simulink library "asbhl20vehicle"  (R2016b)
settings: Solver=ode45  StartTime=0.0  StopTime=10.0  RelTol=1e-3
undefined symbols (not defined in the file): alpha_vec_Cn0, b_ref, beta_vec_Cn0, Clbeta, Clda, Clddf, Cldr, Clp, Clr, Cm0, cm_GE, cm_LG, Cmda, Cmde, Cmdfn, Cmdfp, Cmdr, Cmq, Cn0, Cnda, Cnddf, Cndr, Cnp, Cnr, CX0, cx_GE, cx_LG, CXda, CXddf, CXde, CXdfn, CXdfp, CXdr, CYbeta, CYda, CYddf, CYdr, CZ0, cz_GE, cz_LG, CZda, CZde, CZdfn, CZdfp, CZdr, d_ref, Earth, Euler_0, heading0, LongLat0, mass, Tfg, Tplant, Ts, WGS84, x_cg, x_ref
libraries: aerolibtransform2 x6, aerolibconvert2 x4, aerolibasang x3, aerolibobsolete x3, aerolibutil x3, aerolib6dof2 x1, aerolibadyn x1, asbhl20act x1, discretizing x1
(part 2 of 2)

== system asbhl20vehicle/Vehicle/Aerodynamic/Aerodynamic Coefficients/Actuator Increments/Flap(pos) ==
  Alpha : Inport
  Actuators : Inport  Port=2
  Bus Selector : BusSelector  OutputSignals=Flap(pos)
  Bus Selector1 : BusSelector  OutputSignals=k,f
  Bus Selector3 : BusSelector  OutputSignals=k,f
  Bus Selector5 : BusSelector  OutputSignals=k,f
  Cm : Interpolation_n-D  NumberOfTableDimensions=1  Table=Cmdfp  RemoveProtectionIndex=on  SaturateOnIntegerOverflow=on
      settings: InputPortMap=u0,u1
  Constant1 : Constant  Value=0
  Constant2 : Constant  Value=0
  Constant3 : Constant  Value=0
  Cx : Interpolation_n-D  NumberOfTableDimensions=1  Table=CXdfp  RemoveProtectionIndex=on  SaturateOnIntegerOverflow=on
      settings: InputPortMap=u0,u1
  Cz : Interpolation_n-D  NumberOfTableDimensions=1  Table=CZdfp  RemoveProtectionIndex=on  SaturateOnIntegerOverflow=on
      settings: InputPortMap=u0,u1
  Mux1 : Mux  Inputs=6
  Product : Product  SaturateOnIntegerOverflow=on  InputSameDT=on  OutDataTypeStr=Inherit: Same as first input
  delCoeff : Outport
  wires:
  Product/1 -> delCoeff/1
  Mux1/1 -> Product/1
  Alpha/1 -> Bus Selector5/1, Bus Selector3/1, Bus Selector1/1
  Cx/1 -> Mux1/1
  Cz/1 -> Mux1/3
  Cm/1 -> Mux1/5
  Constant1/1 -> Mux1/2
  Constant2/1 -> Mux1/4
  Constant3/1 -> Mux1/6
  Actuators/1 -> Bus Selector/1
  Bus Selector/1 -> Product/2  "<Flap(pos)>"
  Bus Selector5/1 -> Cm/1  "<k>"
  Bus Selector5/2 -> Cm/2  "<f>"
  Bus Selector3/1 -> Cz/1  "<k>"
  Bus Selector3/2 -> Cz/2  "<f>"
  Bus Selector1/1 -> Cx/1  "<k>"
  Bus Selector1/2 -> Cx/2  "<f>"

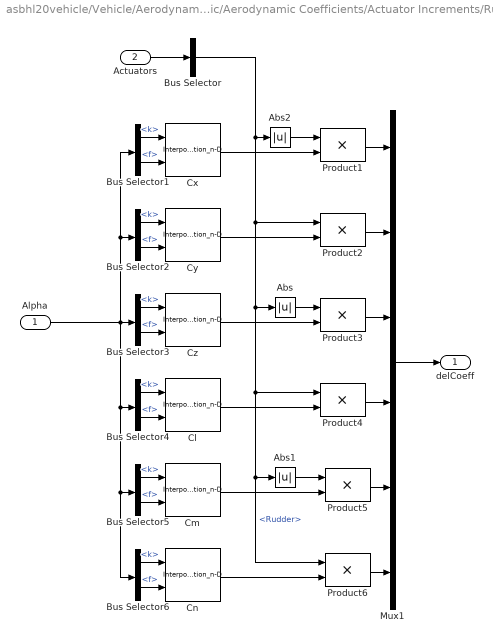
== system asbhl20vehicle/Vehicle/Aerodynamic/Aerodynamic Coefficients/Actuator Increments/Rudder ==
  Alpha : Inport
  Actuators : Inport  Port=2
  Abs : Abs  SaturateOnIntegerOverflow=on
  Abs1 : Abs  SaturateOnIntegerOverflow=on
  Abs2 : Abs  SaturateOnIntegerOverflow=on
  Bus Selector : BusSelector  OutputSignals=Rudder
  Bus Selector{1..6} (6 alike) : BusSelector  OutputSignals=k,f
  Cl : Interpolation_n-D  NumberOfTableDimensions=1  Table=Cldr  RemoveProtectionIndex=on  SaturateOnIntegerOverflow=on
      settings: InputPortMap=u0,u1
  Cm : Interpolation_n-D  NumberOfTableDimensions=1  Table=Cmdr  RemoveProtectionIndex=on  SaturateOnIntegerOverflow=on
      settings: InputPortMap=u0,u1
  Cn : Interpolation_n-D  NumberOfTableDimensions=1  Table=Cndr  RemoveProtectionIndex=on  SaturateOnIntegerOverflow=on
      settings: InputPortMap=u0,u1
  Cx : Interpolation_n-D  NumberOfTableDimensions=1  Table=CXdr  RemoveProtectionIndex=on  SaturateOnIntegerOverflow=on
      settings: InputPortMap=u0,u1
  Cy : Interpolation_n-D  NumberOfTableDimensions=1  Table=CYdr  RemoveProtectionIndex=on  SaturateOnIntegerOverflow=on
      settings: InputPortMap=u0,u1
  Cz : Interpolation_n-D  NumberOfTableDimensions=1  Table=CZdr  RemoveProtectionIndex=on  SaturateOnIntegerOverflow=on
      settings: InputPortMap=u0,u1
  Mux1 : Mux  Inputs=6
  Product{1..6} (6 alike) : Product  SaturateOnIntegerOverflow=on  InputSameDT=on  OutDataTypeStr=Inherit: Same as first input
  delCoeff : Outport
  wires:
  Actuators/1 -> Bus Selector/1
  Mux1/1 -> delCoeff/1
  Product1/1 -> Mux1/1
  Cx/1 -> Product1/2
  Product2/1 -> Mux1/2
  Cy/1 -> Product2/2
  Product3/1 -> Mux1/3
  Cz/1 -> Product3/2
  Cl/1 -> Product4/2
  Product4/1 -> Mux1/4
  Cm/1 -> Product5/2
  Product5/1 -> Mux1/5
  Cn/1 -> Product6/2
  Product6/1 -> Mux1/6
  Bus Selector/1 -> Abs2/1, Product2/1, Abs/1, Product4/1, Abs1/1, Product6/1  "<Rudder>"
  Abs/1 -> Product3/1
  Abs1/1 -> Product5/1
  Abs2/1 -> Product1/1
  Alpha/1 -> Bus Selector3/1, Bus Selector4/1, Bus Selector6/1, Bus Selector5/1, Bus Selector2/1, Bus Selector1/1
  Bus Selector1/1 -> Cx/1  "<k>"
  Bus Selector1/2 -> Cx/2  "<f>"
  Bus Selector2/1 -> Cy/1  "<k>"
  Bus Selector2/2 -> Cy/2  "<f>"
  Bus Selector3/1 -> Cz/1  "<k>"
  Bus Selector3/2 -> Cz/2  "<f>"
  Bus Selector4/1 -> Cl/1  "<k>"
  Bus Selector4/2 -> Cl/2  "<f>"
  Bus Selector5/1 -> Cm/1  "<k>"
  Bus Selector5/2 -> Cm/2  "<f>"
  Bus Selector6/1 -> Cn/1  "<k>"
  Bus Selector6/2 -> Cn/2  "<f>"

== system asbhl20vehicle/Vehicle/Aerodynamic/Aerodynamic Coefficients/Body Rate Damping/p ==
  Alpha : Inport
  Bus Selector : BusSelector  OutputSignals=k,f
  Bus Selector1 : BusSelector  OutputSignals=k,f
  Cl : Interpolation_n-D  NumberOfTableDimensions=1  Table=Clp  RemoveProtectionIndex=on  SaturateOnIntegerOverflow=on
      settings: InputPortMap=u0,u1
  Cn : Interpolation_n-D  NumberOfTableDimensions=1  Table=Cnp  RemoveProtectionIndex=on  SaturateOnIntegerOverflow=on
      settings: InputPortMap=u0,u1
  Constant1 : Constant  Value=0
  Mux1 : Mux  Inputs=6
  delCoeff : Outport
  wires:
  Mux1/1 -> delCoeff/1
  Constant1/1 -> Mux1/1, Mux1/5, Mux1/3, Mux1/2  "Cxp"
  Cn/1 -> Mux1/6
  Cl/1 -> Mux1/4  "Cl"
  Alpha/1 -> Bus Selector/1, Bus Selector1/1
  Bus Selector/1 -> Cl/1  "<k>"
  Bus Selector/2 -> Cl/2  "<f>"
  Bus Selector1/1 -> Cn/1  "<k>"
  Bus Selector1/2 -> Cn/2  "<f>"

== system asbhl20vehicle/Vehicle/Aerodynamic/Aerodynamic Coefficients/Body Rate Damping/q ==
  Alpha : Inport
  Bus Selector1 : BusSelector  OutputSignals=k,f
  Cmq : Interpolation_n-D  NumberOfTableDimensions=1  Table=Cmq  RemoveProtectionIndex=on  SaturateOnIntegerOverflow=on
      settings: InputPortMap=u0,u1
  Constant3 : Constant  Value=0
  Mux1 : Mux  Inputs=6
  delCoeff : Outport
  wires:
  Cmq/1 -> Mux1/5
  Constant3/1 -> Mux1/1, Mux1/2, Mux1/3, Mux1/6, Mux1/4
  Mux1/1 -> delCoeff/1
  Alpha/1 -> Bus Selector1/1
  Bus Selector1/1 -> Cmq/1  "<k>"
  Bus Selector1/2 -> Cmq/2  "<f>"

== system asbhl20vehicle/Vehicle/Aerodynamic/Aerodynamic Coefficients/Body Rate Damping/r ==
  Alpha : Inport
  Bus Selector : BusSelector  OutputSignals=k,f
  Bus Selector1 : BusSelector  OutputSignals=k,f
  Cl : Interpolation_n-D  NumberOfTableDimensions=1  Table=Clr  RemoveProtectionIndex=on  SaturateOnIntegerOverflow=on
      settings: InputPortMap=u0,u1
  Cn : Interpolation_n-D  NumberOfTableDimensions=1  Table=Cnr  RemoveProtectionIndex=on  SaturateOnIntegerOverflow=on
      settings: InputPortMap=u0,u1
  Constant : Constant  Value=0
  Mux1 : Mux  Inputs=6
  delCoeff : Outport
  wires:
  Cn/1 -> Mux1/6
  Cl/1 -> Mux1/4  "Cl"
  Constant/1 -> Mux1/1, Mux1/2, Mux1/5, Mux1/3  "Cxr"
  Mux1/1 -> delCoeff/1
  Alpha/1 -> Bus Selector1/1, Bus Selector/1
  Bus Selector/1 -> Cl/1  "<k>"
  Bus Selector/2 -> Cl/2  "<f>"
  Bus Selector1/1 -> Cn/1  "<k>"
  Bus Selector1/2 -> Cn/2  "<f>"

== system asbhl20vehicle/Vehicle/LandingGear GroundReaction/L Main Gear Geometry Forces and Moments/GenerateGroundFM/Calc Gear Force and Pos ==
  ZrL : Inport
  ZcL : Inport  Port=2
  Xg : Inport  Port=3
  DCM : Inport  Port=4
  Demux1 : Demux  Outputs=3
  Demux2 : Demux  Outputs=3
  Strut Normal Force : Subsystem
  Sum1 : Sum  Inputs=++--
  get_row3 : Selector  NumberOfDimensions=2  InputPortWidth=3  IndexOptions=Index vector (dialog),Select all  Indices=3,-1  OutputSizes=1
  prod1 : Product  RndMeth=Zero
  prod2 : Product  RndMeth=Zero
  dZ_strut : Outport  InitialOutput=0
  Fn_strut : Outport  Port=2  InitialOutput=0
  ZgB_prime : Outport  Port=3  InitialOutput=0
  wires:
  get_row3/1 -> Demux1/1
  Demux1/1 -> prod1/2
  Demux2/1 -> prod1/1
  Sum1/1 -> Strut Normal Force/2(Strut_dZnum)
  Demux1/3 -> Strut Normal Force/3(C33)
  Demux1/2 -> prod2/2
  Demux2/2 -> prod2/1
  Demux2/3 -> Strut Normal Force/1(ZgB)
  ZrL/1 -> Sum1/1
  Strut Normal Force/1(dZ_strut) -> dZ_strut/1
  Strut Normal Force/2(Fn_strut) -> Fn_strut/1
  Xg/1 -> Demux2/1
  DCM/1 -> get_row3/1
  prod2/1 -> Sum1/4
  prod1/1 -> Sum1/3
  ZcL/1 -> Sum1/2
  Strut Normal Force/3(ZgB_prime) -> ZgB_prime/1

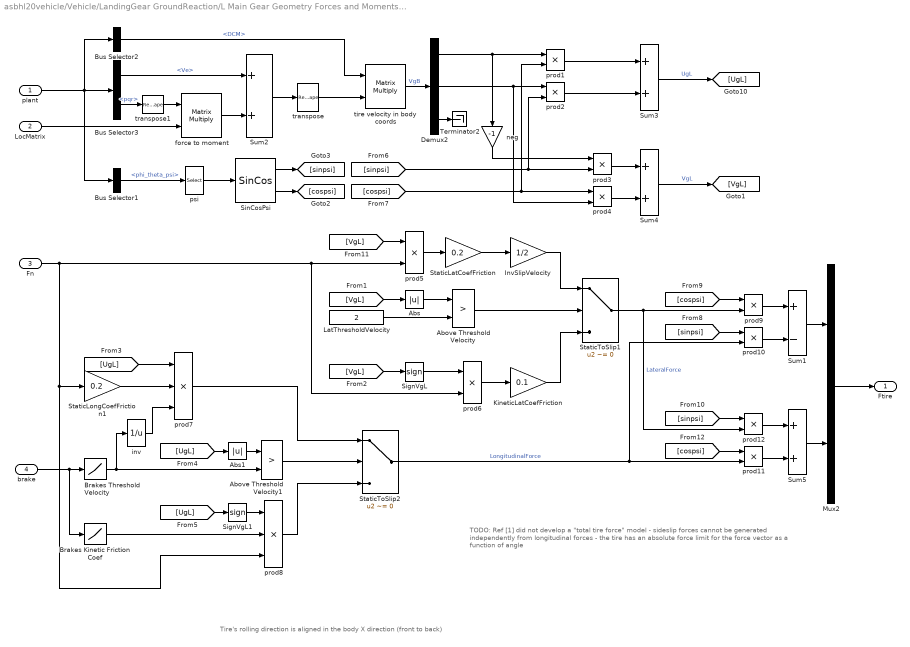
== system asbhl20vehicle/Vehicle/LandingGear GroundReaction/L Main Gear Geometry Forces and Moments/GenerateGroundFM/Calc Tire Force ==
  note: TODO: Ref [1] did not develop a "total tire force" model -
      | sideslip forces cannot be generated independently
      | from longitudinal forces - the tire has an absolute
      | force limit for the force vector as a function of angle
  note: Tire's rolling direction is aligned in the body X direction (front to back)
  plant : Inport
  LocMatrix : Inport  Port=2
  Fn : Inport  Port=3
  brake : Inport  Port=4
  Above Threshold Velocity : RelationalOperator  Operator=>  OutDataTypeStr=boolean  RndMeth=Nearest
  Above Threshold Velocity1 : RelationalOperator  Operator=>  OutDataTypeStr=boolean  RndMeth=Nearest
  Abs : Abs
  Abs1 : Abs
  Brakes Kinetic Friction Coef : Lookup  InputValues=[0 1]  Table=[0.2 0.1]
  Brakes Threshold Velocity : Lookup  InputValues=[0 1]  Table=[2, 50]
  Bus Selector1 : BusSelector  OutputSignals=phi_theta_psi
  Bus Selector2 : BusSelector  OutputSignals=DCM
  Bus Selector3 : BusSelector  OutputSignals=Ve,pqr
  Demux2 : Demux  Outputs=3
  InvSlipVelocity : Gain  Gain=1/2
  KineticLatCoefFriction : Gain  Gain=0.1
  LatThresholdVelocity : Constant  Value=2
  Mux2 : Mux  Inputs=2
  SignVgL : Signum
  SignVgL1 : Signum
  SinCosPsi : aerolibobsolete/SinCos
  StaticLatCoefFriction : Gain  Gain=0.2
  StaticLongCoefFriction1 : Gain  Gain=0.2
  StaticToSlip1 : Switch  Criteria=u2 ~= 0
  StaticToSlip2 : Switch  Criteria=u2 ~= 0
  Sum1 : Sum  Inputs=+-
  Sum2 : Sum  Inputs=2
  Sum3 : Sum  Inputs=2
  Sum4 : Sum  Inputs=2
  Sum5 : Sum
  Terminator2 : Terminator
  force to moment : Product  Multiplication=Matrix(*)  SaturateOnIntegerOverflow=on  InputSameDT=on  OutDataTypeStr=Inherit: Same as first input
  inv : Math  Operator=reciprocal  SaturateOnIntegerOverflow=on
  neg : Gain  Gain=-1
  prod{1..6,9..12} (10 alike) : Product  RndMeth=Zero
  prod7 : Product  Inputs=3  RndMeth=Zero
  prod8 : Product  Inputs=3  RndMeth=Zero
  psi : Selector  InputPortWidth=3  IndexOptions=Index vector (dialog)  Indices=3  OutputSizes=1
  tire velocity in body coords : Product  Multiplication=Matrix(*)  SaturateOnIntegerOverflow=on  InputSameDT=on  OutDataTypeStr=Inherit: Same as first input
  transpose : Reshape  OutputDimensionality=Column vector (2-D)  OutputDimensions=[1,3]
  transpose1 : Reshape  OutputDimensionality=Row vector (2-D)  OutputDimensions=[1,3]
  Ftire : Outport  InitialOutput=0
  wires:
  transpose1/1 -> force to moment/1
  transpose/1 -> tire velocity in body coords/2
  Mux2/1 -> Ftire/1
  Sum5/1 -> Mux2/2
  Sum1/1 -> Mux2/1
  [cospsi] -> prod11/1
  [sinpsi] -> prod12/1
  prod11/1 -> Sum5/2
  prod12/1 -> Sum5/1
  [sinpsi] -> prod10/1
  [cospsi] -> prod9/1
  prod10/1 -> Sum1/2
  prod9/1 -> Sum1/1
  SinCosPsi/2 -> [cospsi]
  SinCosPsi/1 -> [sinpsi]
  psi/1 -> SinCosPsi/1
  StaticToSlip2/1 -> prod11/2, prod10/2  "LongitudinalForce"
  prod8/1 -> StaticToSlip2/3
  Brakes Threshold Velocity/1 -> Above Threshold Velocity1/2, inv/1
  inv/1 -> prod7/3
  SignVgL1/1 -> prod8/1
  [UgL] -> SignVgL1/1
  Above Threshold Velocity1/1 -> StaticToSlip2/2
  Abs1/1 -> Above Threshold Velocity1/1
  [UgL] -> Abs1/1
  prod7/1 -> StaticToSlip2/1
  StaticLongCoefFriction1/1 -> prod7/2
  [UgL] -> prod7/1
  Brakes Kinetic Friction Coef/1 -> prod8/2
  brake/1 -> Brakes Kinetic Friction Coef/1, Brakes Threshold Velocity/1
  StaticToSlip1/1 -> prod12/2, prod9/2  "LateralForce"
  KineticLatCoefFriction/1 -> StaticToSlip1/3
  prod6/1 -> KineticLatCoefFriction/1
  SignVgL/1 -> prod6/1
  [VgL] -> SignVgL/1
  Above Threshold Velocity/1 -> StaticToSlip1/2
  LatThresholdVelocity/1 -> Above Threshold Velocity/2
  Abs/1 -> Above Threshold Velocity/1
  [VgL] -> Abs/1
  InvSlipVelocity/1 -> StaticToSlip1/1
  Fn/1 -> prod8/3, StaticLongCoefFriction1/1, prod6/2, prod5/2
  StaticLatCoefFriction/1 -> InvSlipVelocity/1
  prod5/1 -> StaticLatCoefFriction/1
  [VgL] -> prod5/1
  neg/1 -> prod3/1
  Sum4/1 -> [VgL]  "VgL"
  Sum3/1 -> [UgL]  "UgL"
  prod4/1 -> Sum4/2
  prod3/1 -> Sum4/1
  prod2/1 -> Sum3/2
  prod1/1 -> Sum3/1
  [sinpsi] -> prod3/2, prod2/2
  [cospsi] -> prod4/1, prod1/2
  Demux2/2 -> prod4/2, prod2/1
  Demux2/1 -> neg/1, prod1/1
  Demux2/3 -> Terminator2/1
  tire velocity in body coords/1 -> Demux2/1  "VgB"
  Bus Selector2/1 -> tire velocity in body coords/1  "<DCM>"
  Sum2/1 -> transpose/1
  Bus Selector1/1 -> psi/1  "<phi_theta_psi>"
  Bus Selector3/1 -> Sum2/1  "<Ve>"
  plant/1 -> Bus Selector2/1, Bus Selector1/1, Bus Selector3/1
  force to moment/1 -> Sum2/2
  LocMatrix/1 -> force to moment/2
  Bus Selector3/2 -> transpose1/1  "<pqr>"

== system asbhl20vehicle/Vehicle/LandingGear GroundReaction/L Main Gear Geometry Forces and Moments/GenerateGroundFM/Forces and distances to LMN ==
  Fb : Inport
  Xg_gnd : Inport  Port=2
  force to moment : Product  Multiplication=Matrix(*)  SaturateOnIntegerOverflow=on  InputSameDT=on  OutDataTypeStr=Inherit: Same as first input
  transpose : Reshape  OutputDimensionality=Row vector (2-D)  OutputDimensions=[1,3]
  transpose1 : Reshape  OutputDimensionality=Column vector (2-D)  OutputDimensions=[1,3]
  LMNe : Outport
  wires:
  Fb/1 -> transpose/1
  Xg_gnd/1 -> force to moment/2
  transpose/1 -> force to moment/1
  force to moment/1 -> transpose1/1
  transpose1/1 -> LMNe/1

== system asbhl20vehicle/Vehicle/LandingGear GroundReaction/L Main Gear Geometry Forces and Moments/GenerateGroundFM/LocMatrix ==
  XgB : Inport
  ZgB_prime : Inport  Port=2
  Create 3x3 Matrix : aerolibutil/Create 3x3 Matrix
  Demux2 : Demux  Outputs=3
  Terminator1 : Terminator
  inv1 : Gain  Gain=-1
  inv2 : Gain  Gain=-1
  inv3 : Gain  Gain=-1
  zero1 : Constant  Value=0  SampleTime=0
  zero2 : Constant  Value=0  SampleTime=0
  zero3 : Constant  Value=0  SampleTime=0
  A : Outport
  wires:
  XgB/1 -> Demux2/1
  Demux2/3 -> Terminator1/1
  Demux2/1 -> inv2/1, Create 3x3 Matrix/8
  Demux2/2 -> Create 3x3 Matrix/3, inv3/1
  ZgB_prime/1 -> inv1/1, Create 3x3 Matrix/4
  Create 3x3 Matrix/1 -> A/1
  zero1/1 -> Create 3x3 Matrix/1
  inv1/1 -> Create 3x3 Matrix/2
  zero2/1 -> Create 3x3 Matrix/5
  inv2/1 -> Create 3x3 Matrix/6
  inv3/1 -> Create 3x3 Matrix/7
  zero3/1 -> Create 3x3 Matrix/9

== system asbhl20vehicle/Vehicle/LandingGear GroundReaction/L Main Gear Geometry Forces and Moments/GenerateGroundFM/Subsystem ==
  Euler : Inport
  Bias : Bias  Bias=[0.0 0.0 -heading0*pi/180]
  Rotation Angles to Direction Cosine Matrix : aerolibtransform2/Rotation Angles to Direction Cosine Matrix  rotationOrder=ZYX
  Selector : Selector  InputPortWidth=3  IndexOptions=Index vector (dialog)  Indices=[3 2 1]  OutputSizes=1
  DCM : Outport
  wires:
  Bias/1 -> Selector/1
  Euler/1 -> Bias/1
  Rotation Angles to Direction Cosine Matrix/1 -> DCM/1
  Selector/1 -> Rotation Angles to Direction Cosine Matrix/1

== system asbhl20vehicle/Vehicle/LandingGear GroundReaction/Nose Gear Geometry Forces and Moments/GenerateGroundFM/Calc Gear Force and Pos ==
  ZrL : Inport
  ZcL : Inport  Port=2
  Xg : Inport  Port=3
  DCM : Inport  Port=4
  Demux1 : Demux  Outputs=3
  Demux2 : Demux  Outputs=3
  Strut Normal Force : Subsystem
  Sum1 : Sum  Inputs=++--
  get_row3 : Selector  NumberOfDimensions=2  InputPortWidth=3  IndexOptions=Index vector (dialog),Select all  Indices=3,-1  OutputSizes=1
  prod1 : Product  RndMeth=Zero
  prod2 : Product  RndMeth=Zero
  dZ_strut : Outport  InitialOutput=0
  Fn_strut : Outport  Port=2  InitialOutput=0
  ZgB_prime : Outport  Port=3  InitialOutput=0
  wires:
  get_row3/1 -> Demux1/1
  Demux1/1 -> prod1/2
  Demux2/1 -> prod1/1
  Sum1/1 -> Strut Normal Force/2(Strut_dZnum)
  Demux1/3 -> Strut Normal Force/3(C33)
  Demux1/2 -> prod2/2
  Demux2/2 -> prod2/1
  Demux2/3 -> Strut Normal Force/1(ZgB)
  ZrL/1 -> Sum1/1
  Strut Normal Force/1(dZ_strut) -> dZ_strut/1
  Strut Normal Force/2(Fn_strut) -> Fn_strut/1
  Xg/1 -> Demux2/1
  DCM/1 -> get_row3/1
  prod2/1 -> Sum1/4
  prod1/1 -> Sum1/3
  ZcL/1 -> Sum1/2
  Strut Normal Force/3(ZgB_prime) -> ZgB_prime/1

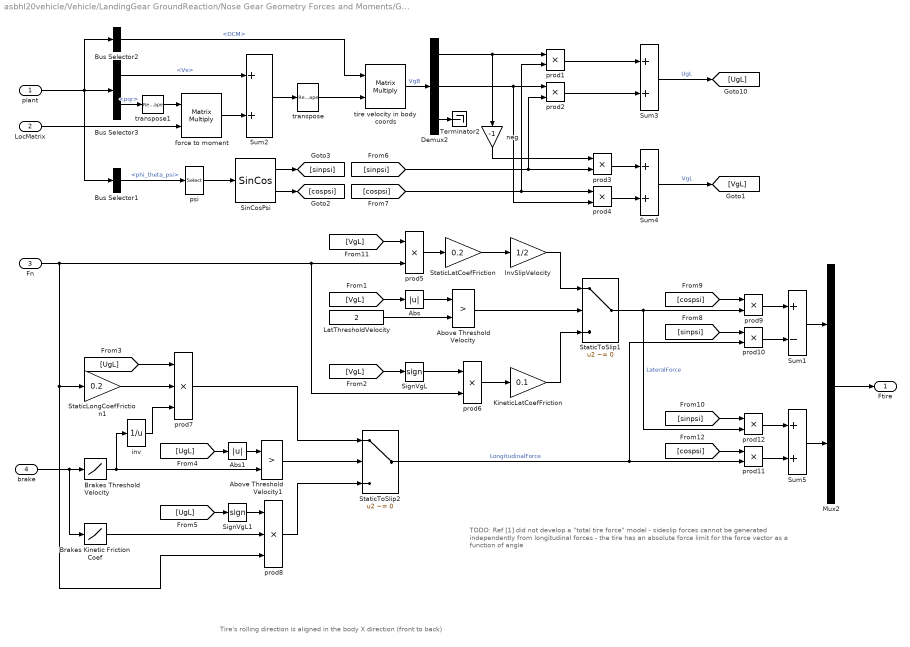
== system asbhl20vehicle/Vehicle/LandingGear GroundReaction/Nose Gear Geometry Forces and Moments/GenerateGroundFM/Calc Tire Force ==
  note: TODO: Ref [1] did not develop a "total tire force" model -
      | sideslip forces cannot be generated independently
      | from longitudinal forces - the tire has an absolute
      | force limit for the force vector as a function of angle
  note: Tire's rolling direction is aligned in the body X direction (front to back)
  plant : Inport
  LocMatrix : Inport  Port=2
  Fn : Inport  Port=3
  brake : Inport  Port=4
  Above Threshold Velocity : RelationalOperator  Operator=>  OutDataTypeStr=boolean  RndMeth=Nearest
  Above Threshold Velocity1 : RelationalOperator  Operator=>  OutDataTypeStr=boolean  RndMeth=Nearest
  Abs : Abs
  Abs1 : Abs
  Brakes Kinetic Friction Coef : Lookup  InputValues=[0 1]  Table=[0.2 0.1]
  Brakes Threshold Velocity : Lookup  InputValues=[0 1]  Table=[2, 50]
  Bus Selector1 : BusSelector  OutputSignals=phi_theta_psi
  Bus Selector2 : BusSelector  OutputSignals=DCM
  Bus Selector3 : BusSelector  OutputSignals=Ve,pqr
  Demux2 : Demux  Outputs=3
  InvSlipVelocity : Gain  Gain=1/2
  KineticLatCoefFriction : Gain  Gain=0.1
  LatThresholdVelocity : Constant  Value=2
  Mux2 : Mux  Inputs=2
  SignVgL : Signum
  SignVgL1 : Signum
  SinCosPsi : aerolibobsolete/SinCos
  StaticLatCoefFriction : Gain  Gain=0.2
  StaticLongCoefFriction1 : Gain  Gain=0.2
  StaticToSlip1 : Switch  Criteria=u2 ~= 0
  StaticToSlip2 : Switch  Criteria=u2 ~= 0
  Sum1 : Sum  Inputs=+-
  Sum2 : Sum  Inputs=2
  Sum3 : Sum  Inputs=2
  Sum4 : Sum  Inputs=2
  Sum5 : Sum
  Terminator2 : Terminator
  force to moment : Product  Multiplication=Matrix(*)  SaturateOnIntegerOverflow=on  InputSameDT=on  OutDataTypeStr=Inherit: Same as first input
  inv : Math  Operator=reciprocal  SaturateOnIntegerOverflow=on
  neg : Gain  Gain=-1
  prod{1..6,9..12} (10 alike) : Product  RndMeth=Zero
  prod7 : Product  Inputs=3  RndMeth=Zero
  prod8 : Product  Inputs=3  RndMeth=Zero
  psi : Selector  InputPortWidth=3  IndexOptions=Index vector (dialog)  Indices=3  OutputSizes=1
  tire velocity in body coords : Product  Multiplication=Matrix(*)  SaturateOnIntegerOverflow=on  InputSameDT=on  OutDataTypeStr=Inherit: Same as first input
  transpose : Reshape  OutputDimensionality=Column vector (2-D)  OutputDimensions=[1,3]
  transpose1 : Reshape  OutputDimensionality=Row vector (2-D)  OutputDimensions=[1,3]
  Ftire : Outport  InitialOutput=0
  wires:
  transpose1/1 -> force to moment/1
  transpose/1 -> tire velocity in body coords/2
  Mux2/1 -> Ftire/1
  Sum5/1 -> Mux2/2
  Sum1/1 -> Mux2/1
  [cospsi] -> prod11/1
  [sinpsi] -> prod12/1
  prod11/1 -> Sum5/2
  prod12/1 -> Sum5/1
  [sinpsi] -> prod10/1
  [cospsi] -> prod9/1
  prod10/1 -> Sum1/2
  prod9/1 -> Sum1/1
  SinCosPsi/2 -> [cospsi]
  SinCosPsi/1 -> [sinpsi]
  psi/1 -> SinCosPsi/1
  StaticToSlip2/1 -> prod11/2, prod10/2  "LongitudinalForce"
  prod8/1 -> StaticToSlip2/3
  Brakes Threshold Velocity/1 -> Above Threshold Velocity1/2, inv/1
  inv/1 -> prod7/3
  SignVgL1/1 -> prod8/1
  [UgL] -> SignVgL1/1
  Above Threshold Velocity1/1 -> StaticToSlip2/2
  Abs1/1 -> Above Threshold Velocity1/1
  [UgL] -> Abs1/1
  prod7/1 -> StaticToSlip2/1
  StaticLongCoefFriction1/1 -> prod7/2
  [UgL] -> prod7/1
  Brakes Kinetic Friction Coef/1 -> prod8/2
  brake/1 -> Brakes Kinetic Friction Coef/1, Brakes Threshold Velocity/1
  StaticToSlip1/1 -> prod12/2, prod9/2  "LateralForce"
  KineticLatCoefFriction/1 -> StaticToSlip1/3
  prod6/1 -> KineticLatCoefFriction/1
  SignVgL/1 -> prod6/1
  [VgL] -> SignVgL/1
  Above Threshold Velocity/1 -> StaticToSlip1/2
  LatThresholdVelocity/1 -> Above Threshold Velocity/2
  Abs/1 -> Above Threshold Velocity/1
  [VgL] -> Abs/1
  InvSlipVelocity/1 -> StaticToSlip1/1
  Fn/1 -> prod8/3, StaticLongCoefFriction1/1, prod6/2, prod5/2
  StaticLatCoefFriction/1 -> InvSlipVelocity/1
  prod5/1 -> StaticLatCoefFriction/1
  [VgL] -> prod5/1
  neg/1 -> prod3/1
  Sum4/1 -> [VgL]  "VgL"
  Sum3/1 -> [UgL]  "UgL"
  prod4/1 -> Sum4/2
  prod3/1 -> Sum4/1
  prod2/1 -> Sum3/2
  prod1/1 -> Sum3/1
  [sinpsi] -> prod3/2, prod2/2
  [cospsi] -> prod4/1, prod1/2
  Demux2/2 -> prod4/2, prod2/1
  Demux2/1 -> neg/1, prod1/1
  Demux2/3 -> Terminator2/1
  tire velocity in body coords/1 -> Demux2/1  "VgB"
  Bus Selector2/1 -> tire velocity in body coords/1  "<DCM>"
  Sum2/1 -> transpose/1
  Bus Selector1/1 -> psi/1  "<phi_theta_psi>"
  Bus Selector3/1 -> Sum2/1  "<Ve>"
  plant/1 -> Bus Selector2/1, Bus Selector1/1, Bus Selector3/1
  force to moment/1 -> Sum2/2
  LocMatrix/1 -> force to moment/2
  Bus Selector3/2 -> transpose1/1  "<pqr>"

== system asbhl20vehicle/Vehicle/LandingGear GroundReaction/Nose Gear Geometry Forces and Moments/GenerateGroundFM/Forces and distances to LMN ==
  Fb : Inport
  Xg_gnd : Inport  Port=2
  force to moment : Product  Multiplication=Matrix(*)  SaturateOnIntegerOverflow=on  InputSameDT=on  OutDataTypeStr=Inherit: Same as first input
  transpose : Reshape  OutputDimensionality=Row vector (2-D)  OutputDimensions=[1,3]
  transpose1 : Reshape  OutputDimensionality=Column vector (2-D)  OutputDimensions=[1,3]
  LMNe : Outport
  wires:
  Fb/1 -> transpose/1
  Xg_gnd/1 -> force to moment/2
  transpose/1 -> force to moment/1
  force to moment/1 -> transpose1/1
  transpose1/1 -> LMNe/1

== system asbhl20vehicle/Vehicle/LandingGear GroundReaction/Nose Gear Geometry Forces and Moments/GenerateGroundFM/LocMatrix ==
  XgB : Inport
  ZgB_prime : Inport  Port=2
  Create 3x3 Matrix : aerolibutil/Create 3x3 Matrix
  Demux2 : Demux  Outputs=3
  Terminator1 : Terminator
  inv1 : Gain  Gain=-1
  inv2 : Gain  Gain=-1
  inv3 : Gain  Gain=-1
  zero1 : Constant  Value=0  SampleTime=0
  zero2 : Constant  Value=0  SampleTime=0
  zero3 : Constant  Value=0  SampleTime=0
  A : Outport
  wires:
  XgB/1 -> Demux2/1
  Demux2/3 -> Terminator1/1
  Demux2/1 -> inv2/1, Create 3x3 Matrix/8
  Demux2/2 -> Create 3x3 Matrix/3, inv3/1
  ZgB_prime/1 -> inv1/1, Create 3x3 Matrix/4
  Create 3x3 Matrix/1 -> A/1
  zero1/1 -> Create 3x3 Matrix/1
  inv1/1 -> Create 3x3 Matrix/2
  zero2/1 -> Create 3x3 Matrix/5
  inv2/1 -> Create 3x3 Matrix/6
  inv3/1 -> Create 3x3 Matrix/7
  zero3/1 -> Create 3x3 Matrix/9

== system asbhl20vehicle/Vehicle/LandingGear GroundReaction/Nose Gear Geometry Forces and Moments/GenerateGroundFM/Subsystem ==
  Euler : Inport
  Bias : Bias  Bias=[0.0 0.0 -heading0*pi/180]
  Rotation Angles to Direction Cosine Matrix : aerolibtransform2/Rotation Angles to Direction Cosine Matrix  rotationOrder=ZYX
  Selector : Selector  InputPortWidth=3  IndexOptions=Index vector (dialog)  Indices=[3 2 1]  OutputSizes=1
  DCM : Outport
  wires:
  Bias/1 -> Selector/1
  Euler/1 -> Bias/1
  Rotation Angles to Direction Cosine Matrix/1 -> DCM/1
  Selector/1 -> Rotation Angles to Direction Cosine Matrix/1

== system asbhl20vehicle/Vehicle/LandingGear GroundReaction/R Main Gear Geometry Forces and Moments/GenerateGroundFM/Calc Gear Force and Pos ==
  ZrL : Inport
  ZcL : Inport  Port=2
  Xg : Inport  Port=3
  DCM : Inport  Port=4
  Demux1 : Demux  Outputs=3
  Demux2 : Demux  Outputs=3
  Strut Normal Force : Subsystem
  Sum1 : Sum  Inputs=++--
  get_row3 : Selector  NumberOfDimensions=2  InputPortWidth=3  IndexOptions=Index vector (dialog),Select all  Indices=3,-1  OutputSizes=1
  prod1 : Product  RndMeth=Zero
  prod2 : Product  RndMeth=Zero
  dZ_strut : Outport  InitialOutput=0
  Fn_strut : Outport  Port=2  InitialOutput=0
  ZgB_prime : Outport  Port=3  InitialOutput=0
  wires:
  Strut Normal Force/3(ZgB_prime) -> ZgB_prime/1
  ZcL/1 -> Sum1/2
  prod1/1 -> Sum1/3
  prod2/1 -> Sum1/4
  DCM/1 -> get_row3/1
  Xg/1 -> Demux2/1
  Strut Normal Force/2(Fn_strut) -> Fn_strut/1
  Strut Normal Force/1(dZ_strut) -> dZ_strut/1
  ZrL/1 -> Sum1/1
  Demux2/3 -> Strut Normal Force/1(ZgB)
  Demux2/2 -> prod2/1
  Demux1/2 -> prod2/2
  Demux1/3 -> Strut Normal Force/3(C33)
  Sum1/1 -> Strut Normal Force/2(Strut_dZnum)
  Demux2/1 -> prod1/1
  Demux1/1 -> prod1/2
  get_row3/1 -> Demux1/1

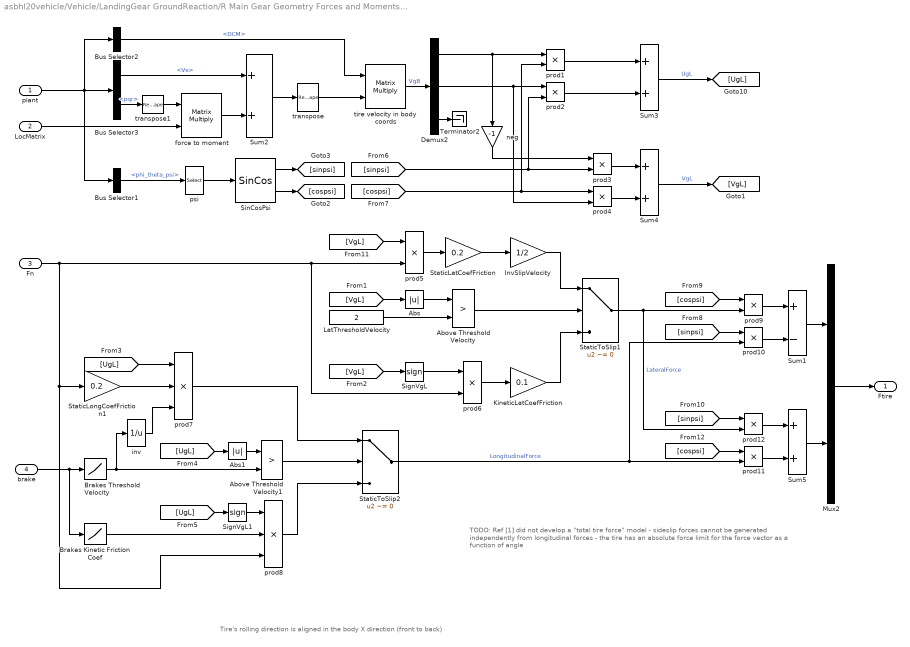
== system asbhl20vehicle/Vehicle/LandingGear GroundReaction/R Main Gear Geometry Forces and Moments/GenerateGroundFM/Calc Tire Force ==
  note: Tire's rolling direction is aligned in the body X direction (front to back)
  note: TODO: Ref [1] did not develop a "total tire force" model -
      | sideslip forces cannot be generated independently
      | from longitudinal forces - the tire has an absolute
      | force limit for the force vector as a function of angle
  plant : Inport
  LocMatrix : Inport  Port=2
  Fn : Inport  Port=3
  brake : Inport  Port=4
  Above Threshold Velocity : RelationalOperator  Operator=>  OutDataTypeStr=boolean  RndMeth=Nearest
  Above Threshold Velocity1 : RelationalOperator  Operator=>  OutDataTypeStr=boolean  RndMeth=Nearest
  Abs : Abs
  Abs1 : Abs
  Brakes Kinetic Friction Coef : Lookup  InputValues=[0 1]  Table=[0.2 0.1]
  Brakes Threshold Velocity : Lookup  InputValues=[0 1]  Table=[2, 50]
  Bus Selector1 : BusSelector  OutputSignals=phi_theta_psi
  Bus Selector2 : BusSelector  OutputSignals=DCM
  Bus Selector3 : BusSelector  OutputSignals=Ve,pqr
  Demux2 : Demux  Outputs=3
  InvSlipVelocity : Gain  Gain=1/2
  KineticLatCoefFriction : Gain  Gain=0.1
  LatThresholdVelocity : Constant  Value=2
  Mux2 : Mux  Inputs=2
  SignVgL : Signum
  SignVgL1 : Signum
  SinCosPsi : aerolibobsolete/SinCos
  StaticLatCoefFriction : Gain  Gain=0.2
  StaticLongCoefFriction1 : Gain  Gain=0.2
  StaticToSlip1 : Switch  Criteria=u2 ~= 0
  StaticToSlip2 : Switch  Criteria=u2 ~= 0
  Sum1 : Sum  Inputs=+-
  Sum2 : Sum  Inputs=2
  Sum3 : Sum  Inputs=2
  Sum4 : Sum  Inputs=2
  Sum5 : Sum
  Terminator2 : Terminator
  force to moment : Product  Multiplication=Matrix(*)  SaturateOnIntegerOverflow=on  InputSameDT=on  OutDataTypeStr=Inherit: Same as first input
  inv : Math  Operator=reciprocal  SaturateOnIntegerOverflow=on
  neg : Gain  Gain=-1
  prod{1..6,9..12} (10 alike) : Product  RndMeth=Zero
  prod7 : Product  Inputs=3  RndMeth=Zero
  prod8 : Product  Inputs=3  RndMeth=Zero
  psi : Selector  InputPortWidth=3  IndexOptions=Index vector (dialog)  Indices=3  OutputSizes=1
  tire velocity in body coords : Product  Multiplication=Matrix(*)  SaturateOnIntegerOverflow=on  InputSameDT=on  OutDataTypeStr=Inherit: Same as first input
  transpose : Reshape  OutputDimensionality=Column vector (2-D)  OutputDimensions=[1,3]
  transpose1 : Reshape  OutputDimensionality=Row vector (2-D)  OutputDimensions=[1,3]
  Ftire : Outport  InitialOutput=0
  wires:
  Bus Selector3/2 -> transpose1/1  "<pqr>"
  LocMatrix/1 -> force to moment/2
  force to moment/1 -> Sum2/2
  plant/1 -> Bus Selector3/1, Bus Selector1/1, Bus Selector2/1
  Bus Selector3/1 -> Sum2/1  "<Ve>"
  Bus Selector1/1 -> psi/1  "<phi_theta_psi>"
  Sum2/1 -> transpose/1
  Bus Selector2/1 -> tire velocity in body coords/1  "<DCM>"
  tire velocity in body coords/1 -> Demux2/1  "VgB"
  Demux2/3 -> Terminator2/1
  Demux2/1 -> prod1/1, neg/1
  Demux2/2 -> prod2/1, prod4/2
  [cospsi] -> prod1/2, prod4/1
  [sinpsi] -> prod2/2, prod3/2
  prod1/1 -> Sum3/1
  prod2/1 -> Sum3/2
  prod3/1 -> Sum4/1
  prod4/1 -> Sum4/2
  Sum3/1 -> [UgL]  "UgL"
  Sum4/1 -> [VgL]  "VgL"
  neg/1 -> prod3/1
  [VgL] -> prod5/1
  prod5/1 -> StaticLatCoefFriction/1
  StaticLatCoefFriction/1 -> InvSlipVelocity/1
  Fn/1 -> prod5/2, prod6/2, StaticLongCoefFriction1/1, prod8/3
  InvSlipVelocity/1 -> StaticToSlip1/1
  [VgL] -> Abs/1
  Abs/1 -> Above Threshold Velocity/1
  LatThresholdVelocity/1 -> Above Threshold Velocity/2
  Above Threshold Velocity/1 -> StaticToSlip1/2
  [VgL] -> SignVgL/1
  SignVgL/1 -> prod6/1
  prod6/1 -> KineticLatCoefFriction/1
  KineticLatCoefFriction/1 -> StaticToSlip1/3
  StaticToSlip1/1 -> prod9/2, prod12/2  "LateralForce"
  brake/1 -> Brakes Threshold Velocity/1, Brakes Kinetic Friction Coef/1
  Brakes Kinetic Friction Coef/1 -> prod8/2
  [UgL] -> prod7/1
  StaticLongCoefFriction1/1 -> prod7/2
  prod7/1 -> StaticToSlip2/1
  [UgL] -> Abs1/1
  Abs1/1 -> Above Threshold Velocity1/1
  Above Threshold Velocity1/1 -> StaticToSlip2/2
  [UgL] -> SignVgL1/1
  SignVgL1/1 -> prod8/1
  inv/1 -> prod7/3
  Brakes Threshold Velocity/1 -> inv/1, Above Threshold Velocity1/2
  prod8/1 -> StaticToSlip2/3
  StaticToSlip2/1 -> prod10/2, prod11/2  "LongitudinalForce"
  psi/1 -> SinCosPsi/1
  SinCosPsi/1 -> [sinpsi]
  SinCosPsi/2 -> [cospsi]
  prod9/1 -> Sum1/1
  prod10/1 -> Sum1/2
  [cospsi] -> prod9/1
  [sinpsi] -> prod10/1
  prod12/1 -> Sum5/1
  prod11/1 -> Sum5/2
  [sinpsi] -> prod12/1
  [cospsi] -> prod11/1
  Sum1/1 -> Mux2/1
  Sum5/1 -> Mux2/2
  Mux2/1 -> Ftire/1
  transpose/1 -> tire velocity in body coords/2
  transpose1/1 -> force to moment/1

== system asbhl20vehicle/Vehicle/LandingGear GroundReaction/R Main Gear Geometry Forces and Moments/GenerateGroundFM/Forces and distances to LMN ==
  Fb : Inport
  Xg_gnd : Inport  Port=2
  force to moment : Product  Multiplication=Matrix(*)  SaturateOnIntegerOverflow=on  InputSameDT=on  OutDataTypeStr=Inherit: Same as first input
  transpose : Reshape  OutputDimensionality=Row vector (2-D)  OutputDimensions=[1,3]
  transpose1 : Reshape  OutputDimensionality=Column vector (2-D)  OutputDimensions=[1,3]
  LMNe : Outport
  wires:
  transpose1/1 -> LMNe/1
  force to moment/1 -> transpose1/1
  transpose/1 -> force to moment/1
  Xg_gnd/1 -> force to moment/2
  Fb/1 -> transpose/1

== system asbhl20vehicle/Vehicle/LandingGear GroundReaction/R Main Gear Geometry Forces and Moments/GenerateGroundFM/LocMatrix ==
  XgB : Inport
  ZgB_prime : Inport  Port=2
  Create 3x3 Matrix : aerolibutil/Create 3x3 Matrix
  Demux2 : Demux  Outputs=3
  Terminator1 : Terminator
  inv1 : Gain  Gain=-1
  inv2 : Gain  Gain=-1
  inv3 : Gain  Gain=-1
  zero1 : Constant  Value=0  SampleTime=0
  zero2 : Constant  Value=0  SampleTime=0
  zero3 : Constant  Value=0  SampleTime=0
  A : Outport
  wires:
  zero3/1 -> Create 3x3 Matrix/9
  inv3/1 -> Create 3x3 Matrix/7
  inv2/1 -> Create 3x3 Matrix/6
  zero2/1 -> Create 3x3 Matrix/5
  inv1/1 -> Create 3x3 Matrix/2
  zero1/1 -> Create 3x3 Matrix/1
  Create 3x3 Matrix/1 -> A/1
  ZgB_prime/1 -> Create 3x3 Matrix/4, inv1/1
  Demux2/2 -> inv3/1, Create 3x3 Matrix/3
  Demux2/1 -> Create 3x3 Matrix/8, inv2/1
  Demux2/3 -> Terminator1/1
  XgB/1 -> Demux2/1

== system asbhl20vehicle/Vehicle/LandingGear GroundReaction/R Main Gear Geometry Forces and Moments/GenerateGroundFM/Subsystem ==
  Euler : Inport
  Bias : Bias  Bias=[0.0 0.0 -heading0*pi/180]
  Rotation Angles to Direction Cosine Matrix : aerolibtransform2/Rotation Angles to Direction Cosine Matrix  rotationOrder=ZYX
  Selector : Selector  InputPortWidth=3  IndexOptions=Index vector (dialog)  Indices=[3 2 1]  OutputSizes=1
  DCM : Outport
  wires:
  Bias/1 -> Selector/1
  Euler/1 -> Bias/1
  Rotation Angles to Direction Cosine Matrix/1 -> DCM/1
  Selector/1 -> Rotation Angles to Direction Cosine Matrix/1

== system asbhl20vehicle/Vehicle/LandingGear GroundReaction/L Main Gear Geometry Forces and Moments/GenerateGroundFM/Calc Gear Force and Pos/Strut Normal Force ==
  note: This derivative is not the same
      | as the one used in reference [1]
  ZgB : Inport
  Strut_dZnum : Inport  Port=2
  C33 : Inport  Port=3
  ComprRate : Gain  Gain=1/Tfg
  DampingRate_N/m/sec : Gain  Gain=1e5
  NormalForce : Product  Inputs=*/  RndMeth=Zero
  RangeLimit : Saturate  LowerLimit=0
  SpringRate_N/m : Gain  Gain=1e5
  Sum1 : Sum  Inputs=+-
  Sum2 : Sum
  Xcmpr_prev : Memory  InheritSampleTime=on
  compression : Product  Inputs=*/  RndMeth=Zero
  dCompression : Sum  Inputs=+-
  ground only pushes : Saturate  UpperLimit=inf  LowerLimit=0
  reaction : Gain  Gain=-1
  dZ_strut : Outport
  Fn_strut : Outport  Port=2
  ZgB_prime : Outport  Port=3
  wires:
  Sum2/1 -> NormalForce/1  "Fstrut"
  RangeLimit/1 -> Xcmpr_prev/1, dCompression/1, dZ_strut/1, SpringRate_N/m/1
  ComprRate/1 -> DampingRate_N/m/sec/1
  SpringRate_N/m/1 -> Sum2/1
  DampingRate_N/m/sec/1 -> Sum2/2
  dCompression/1 -> ComprRate/1
  Xcmpr_prev/1 -> dCompression/2
  Strut_dZnum/1 -> compression/1
  C33/1 -> compression/2, NormalForce/2
  NormalForce/1 -> ground only pushes/1
  ZgB/1 -> Sum1/1
  compression/1 -> Sum1/2, ZgB_prime/1
  Sum1/1 -> RangeLimit/1
  ground only pushes/1 -> reaction/1
  reaction/1 -> Fn_strut/1

== system asbhl20vehicle/Vehicle/LandingGear GroundReaction/Nose Gear Geometry Forces and Moments/GenerateGroundFM/Calc Gear Force and Pos/Strut Normal Force ==
  note: This derivative is not the same
      | as the one used in reference [1]
  ZgB : Inport
  Strut_dZnum : Inport  Port=2
  C33 : Inport  Port=3
  ComprRate : Gain  Gain=1/Tfg
  DampingRate_N/m/sec : Gain  Gain=1e5
  NormalForce : Product  Inputs=*/  RndMeth=Zero
  RangeLimit : Saturate  LowerLimit=0
  SpringRate_N/m : Gain  Gain=1e5
  Sum1 : Sum  Inputs=+-
  Sum2 : Sum
  Xcmpr_prev : Memory  InheritSampleTime=on
  compression : Product  Inputs=*/  RndMeth=Zero
  dCompression : Sum  Inputs=+-
  ground only pushes : Saturate  UpperLimit=inf  LowerLimit=0
  reaction : Gain  Gain=-1
  dZ_strut : Outport
  Fn_strut : Outport  Port=2
  ZgB_prime : Outport  Port=3
  wires:
  Sum2/1 -> NormalForce/1  "Fstrut"
  RangeLimit/1 -> Xcmpr_prev/1, dCompression/1, dZ_strut/1, SpringRate_N/m/1
  ComprRate/1 -> DampingRate_N/m/sec/1
  SpringRate_N/m/1 -> Sum2/1
  DampingRate_N/m/sec/1 -> Sum2/2
  dCompression/1 -> ComprRate/1
  Xcmpr_prev/1 -> dCompression/2
  Strut_dZnum/1 -> compression/1
  C33/1 -> compression/2, NormalForce/2
  NormalForce/1 -> ground only pushes/1
  ZgB/1 -> Sum1/1
  compression/1 -> Sum1/2, ZgB_prime/1
  Sum1/1 -> RangeLimit/1
  ground only pushes/1 -> reaction/1
  reaction/1 -> Fn_strut/1

== system asbhl20vehicle/Vehicle/LandingGear GroundReaction/R Main Gear Geometry Forces and Moments/GenerateGroundFM/Calc Gear Force and Pos/Strut Normal Force ==
  note: This derivative is not the same
      | as the one used in reference [1]
  ZgB : Inport
  Strut_dZnum : Inport  Port=2
  C33 : Inport  Port=3
  ComprRate : Gain  Gain=1/Tfg
  DampingRate_N/m/sec : Gain  Gain=1e5
  NormalForce : Product  Inputs=*/  RndMeth=Zero
  RangeLimit : Saturate  LowerLimit=0
  SpringRate_N/m : Gain  Gain=1e5
  Sum1 : Sum  Inputs=+-
  Sum2 : Sum
  Xcmpr_prev : Memory  InheritSampleTime=on
  compression : Product  Inputs=*/  RndMeth=Zero
  dCompression : Sum  Inputs=+-
  ground only pushes : Saturate  UpperLimit=inf  LowerLimit=0
  reaction : Gain  Gain=-1
  dZ_strut : Outport
  Fn_strut : Outport  Port=2
  ZgB_prime : Outport  Port=3
  wires:
  reaction/1 -> Fn_strut/1
  ground only pushes/1 -> reaction/1
  Sum1/1 -> RangeLimit/1
  compression/1 -> ZgB_prime/1, Sum1/2
  ZgB/1 -> Sum1/1
  NormalForce/1 -> ground only pushes/1
  C33/1 -> NormalForce/2, compression/2
  Strut_dZnum/1 -> compression/1
  Xcmpr_prev/1 -> dCompression/2
  dCompression/1 -> ComprRate/1
  DampingRate_N/m/sec/1 -> Sum2/2
  SpringRate_N/m/1 -> Sum2/1
  ComprRate/1 -> DampingRate_N/m/sec/1
  RangeLimit/1 -> SpringRate_N/m/1, dZ_strut/1, dCompression/1, Xcmpr_prev/1
  Sum2/1 -> NormalForce/1  "Fstrut"
